simulink model "programmer"  (Simulink 7.6)
settings: Solver=FixedStepDiscrete  StartTime=0.0  StopTime=10.0  FixedStep=1  RelTol=1e-3
settings Model: Creator=jordan  LastModifiedBy=jordan
settings DataIOCC: LimitDataPoints=off  SaveOutput=off  SignalLogging=off  DSMLogging=off  SaveTime=off
settings OptimizationCC: BlockReduction=off  ConditionallyExecuteInputs=off

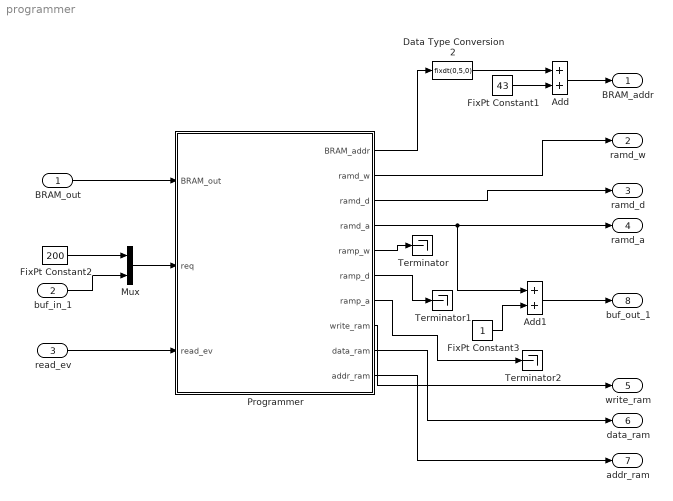
== system programmer ==
  BRAM_out : Inport  OutDataTypeStr=uint8
  buf_in_1 : Inport  Port=2  OutDataTypeStr=uint8  PortDimensions=2
  read_ev : Inport  Port=3
  Add : Sum  AccumDataTypeStr=fixdt(0,11,0)  OutDataTypeStr=fixdt(0,11,0)
  Add1 : Sum  AccumDataTypeStr=uint16  OutDataTypeStr=uint16
  Data Type Conversion2 : DataTypeConversion  OutDataTypeStr=fixdt(0,5,0)
  FixPt Constant1 : Constant  DisableCoverage=on  Value=43  OutDataTypeStr=fixdt(0,11,0)
  FixPt Constant2 : Constant  DisableCoverage=on  Value=200  OutDataTypeStr=uint8
  FixPt Constant3 : Constant  DisableCoverage=on  OutDataTypeStr=fixdt(0,12,0)
  Mux : Mux  Inputs=2
  Programmer : Stateflow chart  TreatAsAtomicUnit=on
  Terminator : Terminator
  Terminator1 : Terminator
  Terminator2 : Terminator
  BRAM_addr : Outport
  ramd_w : Outport  Port=2
  ramd_d : Outport  Port=3
  ramd_a : Outport  Port=4
  write_ram : Outport  Port=5
  data_ram : Outport  Port=6
  addr_ram : Outport  Port=7
  buf_out_1 : Outport  Port=8
  wires:
  Add/1 -> BRAM_addr/1
  FixPt Constant1/1 -> Add/2
  Data Type Conversion2/1 -> Add/1
  Programmer/1(BRAM_addr) -> Data Type Conversion2/1
  Mux/1 -> Programmer/2(req)
  FixPt Constant2/1 -> Mux/1
  buf_in_1/1 -> Mux/2
  Programmer/4(ramd_a) -> Add1/1, ramd_a/1
  Add1/1 -> buf_out_1/1
  Programmer/2(ramd_w) -> ramd_w/1
  Programmer/3(ramd_d) -> ramd_d/1
  Programmer/8(write_ram) -> write_ram/1
  Programmer/9(data_ram) -> data_ram/1
  Programmer/10(addr_ram) -> addr_ram/1
  BRAM_out/1 -> Programmer/1(BRAM_out)
  FixPt Constant3/1 -> Add1/2
  Programmer/5(ramp_w) -> Terminator/1
  Programmer/6(ramp_d) -> Terminator1/1
  Programmer/7(ramp_a) -> Terminator2/1
  read_ev/1 -> Programmer/3(read_ev)

== stateflow chart Programmer ==
  settings: executeAtInitialization=1
  state Start
  state Ready
  state Request
  state Data
  state Wait
  state End
  state Wait1
  state Ready1
  state Data1
  state Data2
  state Data3
  state End1
  (default) -> Start
  Start -> Wait1 : {addr_ram=0;
      | data_ram=100;
      | write_ram=1;
      | ramd_a=0;}
  Ready -> Ready1 : [read_ev]{BRAM_addr=0;}
  Request -> Data1 : {addr_ram=ind;
      | data_ram=req[ind];
      | write_ram=1;}
  (junction 15) -> (junction 18) [order 1] : [BRAM_out==101]
  (junction 15) -> Ready [order 2]
  (junction 16) -> Request [order 2] : {ind++;}
  Data1 -> (junction 16)
  Ready1 -> (junction 15)
  Wait1 -> Ready : {write_ram=0;}
  (junction 16) -> Wait [order 1] : [ind==2]
  Data3 -> (junction 22) : {ramd_w=0;}
  Wait -> Data : [read_ev]{BRAM_addr=0;}
  Data -> (junction 17)
  (junction 18) -> Request : {ind=0;}
  (junction 17) -> (junction 19) [order 2]
  (junction 19) -> (junction 18) : {ramd_a++;}
  (junction 17) -> Data2 [order 1] : [BRAM_out==201]{
      | ind=0;
      | BRAM_addr=1;}
  Data2 -> (junction 20) : {ramd_d[ind]=BRAM_out;
      | ind++;
      | BRAM_addr++;}
  (junction 20) -> (junction 21) [order 2]
  (junction 21) -> Data2
  (junction 20) -> Data3 [order 1] : [ind==3]{
      | ramd_w=1;}
  (junction 22) -> End [order 1] : [ramd_a==2048]{
      | addr_ram=0;
      | data_ram=300;
      | write_ram=1;}
  (junction 22) -> (junction 19) [order 2]
  End -> End1 : {write_ram=0;}
  data: BRAM_out input uint8 size=1; BRAM_addr output fixdt(0,2,0) =0; ramd_w output boolean; ramd_d output uint8 size=4; ramd_a output fixdt(0,12,0); ramp_w output boolean; ramp_d output uint8 size=4; ramp_a output fixdt(0,12,0); write_ram output boolean; data_ram output uint8; addr_ram output fixdt(0,14,0); req input uint8 size=3; ind local uint16; read_ev input boolean
